simulink library "Simple_House_ISOgm_CONF"  (Simulink 8.2)
settings: Solver=ode45  StartTime=0.0  StopTime=10.0  RelTol=1e-3
libraries: carnot x1
settings Model: Creator=lena.frank  LastModifiedBy=drhf

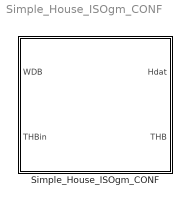
== system Simple_House_ISOgm_CONF ==
  Simple_House_ISOgm_CONF : Subsystem  mask(Simple House with ISO 13370 Ground Model){parameterfile=Default_SimpleHouseISOgm, tini=20}
      mask prompts: parameterfile "Parameter set"; tini "Initial temperature in °C"
      mask help: Preconfigurated parameter sets.
      mask init:
      | % path definitions
      | intpath = fullfile(path_carnot('intlibsl'), ...
      |     'Load','Houses','Simple_House_ISOgm_CONF','parameter_set');
      | pubpath = fullfile(path_carnot('libsl'), ...
      |     'Load','Houses','Simple_House_ISOgm_CONF','parameter_set');
      | 
      | [namelist, lib] = CarnotCallbacks_getConfNamelist(intpath,pubpath);
      | 
      | if ~lib
      |     myMaskStylesVar{1} = ['popup(', namelist,')'];
      |     myMaskStylesVar{2} = 'edit';
      |     set_param(gcb, 'MaskStyles', myMaskStylesVar)
      | end
      | 
      | if exist(fullfile(intpath,[parameterfile '.mat']))
      |     load(fullfile(intpath,parameterfile));
      | else
      |     load(fullfile(pubpath,parameterfile));
      | end
      mask Help: web(fullfile(path_carnot('help'),'simple_house.html'),'-helpbrowser')
      mask TypeOptions parameterfile: Default_SimpleHouseISOgm
      mask Display:
      | % user defined picture file
      | picfile = fullfile(path_carnot('intlibsl'), ...
      |         'Load','Houses','Simple_House_ISOgm_CONF','parameter_set', ...
      |         'Simple_House_ISOgm_CONF.jpg');
      | 
      | % show internal picture if defined
      | if ~BlockIsInCarnotLibrary ...      % if not located in library any more
      |         && exist(picfile,'file')    % AND picfile is present
      |     image(imread(picfile), [0.15 0.1 0.7 0.8])
      |     set_param(gcb, 'BackgroundColor', 'White')
      | else
      |     % show public picture
      |     plot([10,10,90,90,10]/100,[0,50,50,0,0]/100,...
      |          [100,60,40,0]/100,[40,80,80,40]/100,...
      |          [20,34,34,20,20]/100,[40,40,20,20,40]/100,...
      |          [60,60,40,40]/100,[0,40,40,0]/100,...
      |          [65,80,80,65,65]/100,[40,40,20,20,40]/100,...
      |          [47,54,54,47,47]/100,[35,35,4,4,35]/100,...
      |          [45,41]/100,[20,20]/100)
      |     set_param(gcb, 'BackgroundColor', 'Orange')
      | end
      | 
      | % port labels
      | port_label('input',1,'WDB')
      | port_label('input',2,'THB')
      | port_label('output',1,'Hdat')
      | port_label('output',2,'THB')

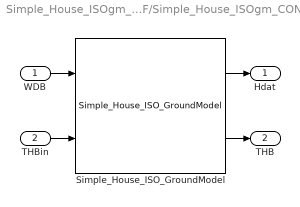
== system Simple_House_ISOgm_CONF/Simple_House_ISOgm_CONF ==
  WDB : Inport
  THBin : Inport  Port=2
  Simple_House_ISO_GroundModel : carnot/Load/Houses/Simple_House_ISO_GroundModel  Ahabit=SH.Ahabit  Hroom=SH.Hroom  Floorsize=SH.Slab  UAwall=SH.UAwall  UAneighbour=0  Uground=0.2  mc=SH.cap  Awin=SH.Awindow  AziWin=SH.AziWindow  Uwin=SH.Uwindow  Gwin=SH.Gwindow  shade=SH.shading  tini=tini  vent=SH.Ventilationrate  rec=SH.Heatrecovery  uaheating=SH.UAheatingsystem  dpcoeff=SH.DpHeatingsystem  heatload=SH.Heatload  delta_t_nom=SH.DTnomHeatingsystem  n_rad=SH.RadiatorExponent  mass_times_cap=SH.CapHeatingsystem
  Hdat : Outport
  THB : Outport  Port=2
  wires:
  Simple_House_ISO_GroundModel/2 -> THB/1
  THBin/1 -> Simple_House_ISO_GroundModel/2
  Simple_House_ISO_GroundModel/1 -> Hdat/1
  WDB/1 -> Simple_House_ISO_GroundModel/1
